simulink subsystem "canStates"  (R2022b)
settings: Solver=VariableStepAuto  StartTime=0.0  StopTime=10.0  RelTol=1e-3
libraries: states_lib x32
settings Model: Creator=serga  LastModifiedBy=serga

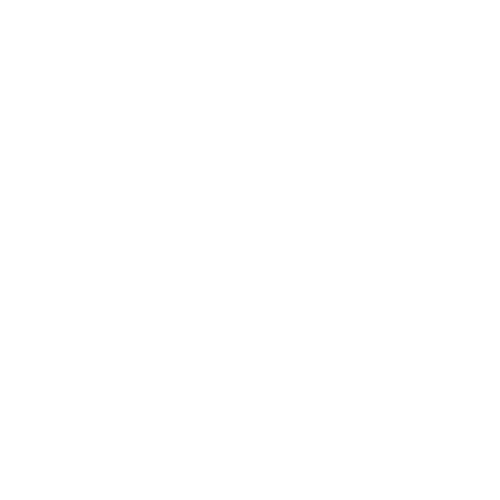
[thumbnail: Simulink's stored preview of the top-level diagram]
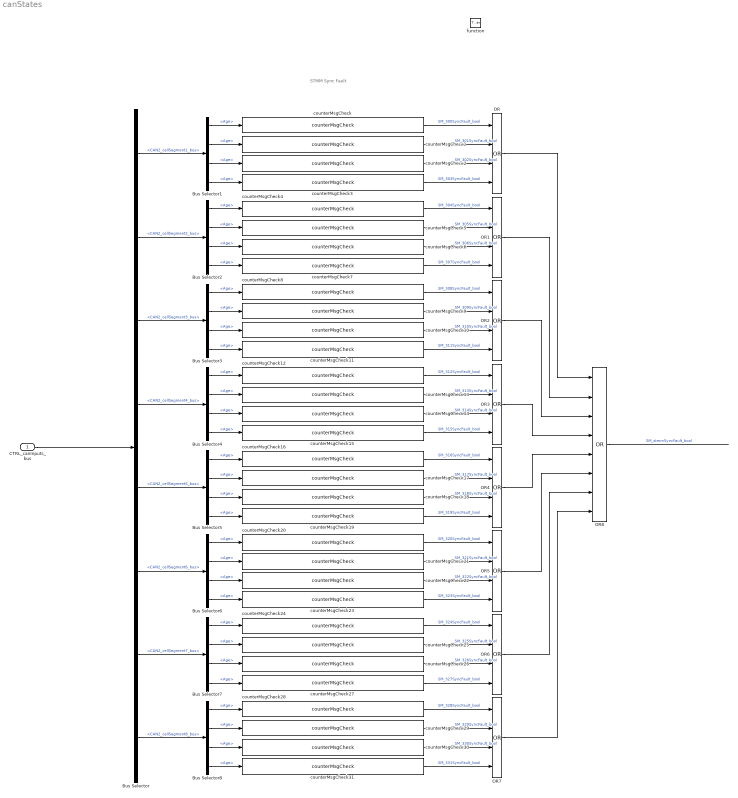
== system canStates ==
  note: STMM Sync Fault
  CTRL_canInputs_bus : Inport
  function : TriggerPort  TriggerType=function-call  VariantControl=(inherit)
  Bus Selector : BusSelector  OutputSignals=IN_can2Inputs_bus.CAN2_stmm_bus.CAN2_cellSegment1_bus,IN_can2Inputs_bus.CAN2_stmm_bus.CAN2_cellSegment2_bus,IN_can2Inputs_bus.CAN2_stmm_bus.CAN2_cellSegment3_bus,IN_can2Inputs_bus.CAN2_stmm_bus.CAN2_cellSegment4_bus,IN_can2Inputs_bus.CAN2_stmm_bus.CAN2_cellSegment5_bus,IN_can2Inputs_bus.CAN2_stmm_bus.CAN2_cellSegment6_bus,IN_can2Inputs_bus.CAN2_stmm_bus.CAN2_cellSegment7_bus,IN_can2Inputs_bus.CAN2_stmm_bus.CAN2_cellSegment8_bus
  Bus Selector1 : BusSelector  OutputSignals=CAN2_stmm_300_bus.Age,CAN2_stmm_301_bus.Age,CAN2_stmm_302_bus.Age,CAN2_stmm_303_bus.Age
  Bus Selector2 : BusSelector  OutputSignals=CAN2_stmm_304_bus.Age,CAN2_stmm_305_bus.Age,CAN2_stmm_306_bus.Age,CAN2_stmm_307_bus.Age
  Bus Selector3 : BusSelector  OutputSignals=CAN2_stmm_308_bus.Age,CAN2_stmm_309_bus.Age,CAN2_stmm_310_bus.Age,CAN2_stmm_311_bus.Age
  Bus Selector4 : BusSelector  OutputSignals=CAN2_stmm_312_bus.Age,CAN2_stmm_313_bus.Age,CAN2_stmm_314_bus.Age,CAN2_stmm_315_bus.Age
  Bus Selector5 : BusSelector  OutputSignals=CAN2_stmm_316_bus.Age,CAN2_stmm_317_bus.Age,CAN2_stmm_318_bus.Age,CAN2_stmm_319_bus.Age
  Bus Selector6 : BusSelector  OutputSignals=CAN2_stmm_320_bus.Age,CAN2_stmm_321_bus.Age,CAN2_stmm_322_bus.Age,CAN2_stmm_323_bus.Age
  Bus Selector7 : BusSelector  OutputSignals=CAN2_stmm_324_bus.Age,CAN2_stmm_325_bus.Age,CAN2_stmm_326_bus.Age,CAN2_stmm_327_bus.Age
  Bus Selector8 : BusSelector  OutputSignals=CAN2_stmm_328_bus.Age,CAN2_stmm_329_bus.Age,CAN2_stmm_330_bus.Age,CAN2_stmm_331_bus.Age
  OR{,1..7} (8 alike) : Logic  Operator=OR  Inputs=4  IconShape=distinctive  AllPortsSameDT=off  OutDataTypeStr=boolean
  OR8 : Logic  Operator=OR  Inputs=8  IconShape=distinctive  AllPortsSameDT=off  OutDataTypeStr=boolean
  counterMsgCheck : states_lib/counterMsgCheck  pos='300'
  counterMsgCheck1 : states_lib/counterMsgCheck  pos='301'
  counterMsgCheck10 : states_lib/counterMsgCheck  pos='310'
  counterMsgCheck11 : states_lib/counterMsgCheck  pos='311'
  counterMsgCheck12 : states_lib/counterMsgCheck  pos='312'
  counterMsgCheck13 : states_lib/counterMsgCheck  pos='313'
  counterMsgCheck14 : states_lib/counterMsgCheck  pos='314'
  counterMsgCheck15 : states_lib/counterMsgCheck  pos='315'
  counterMsgCheck16 : states_lib/counterMsgCheck  pos='316'
  counterMsgCheck17 : states_lib/counterMsgCheck  pos='317'
  counterMsgCheck18 : states_lib/counterMsgCheck  pos='318'
  counterMsgCheck19 : states_lib/counterMsgCheck  pos='319'
  counterMsgCheck2 : states_lib/counterMsgCheck  pos='302'
  counterMsgCheck20 : states_lib/counterMsgCheck  pos='320'
  counterMsgCheck21 : states_lib/counterMsgCheck  pos='321'
  counterMsgCheck22 : states_lib/counterMsgCheck  pos='322'
  counterMsgCheck23 : states_lib/counterMsgCheck  pos='323'
  counterMsgCheck24 : states_lib/counterMsgCheck  pos='324'
  counterMsgCheck25 : states_lib/counterMsgCheck  pos='325'
  counterMsgCheck26 : states_lib/counterMsgCheck  pos='326'
  counterMsgCheck27 : states_lib/counterMsgCheck  pos='327'
  counterMsgCheck28 : states_lib/counterMsgCheck  pos='328'
  counterMsgCheck29 : states_lib/counterMsgCheck  pos='329'
  counterMsgCheck3 : states_lib/counterMsgCheck  pos='303'
  counterMsgCheck30 : states_lib/counterMsgCheck  pos='330'
  counterMsgCheck31 : states_lib/counterMsgCheck  pos='331'
  counterMsgCheck4 : states_lib/counterMsgCheck  pos='304'
  counterMsgCheck5 : states_lib/counterMsgCheck  pos='305'
  counterMsgCheck6 : states_lib/counterMsgCheck  pos='306'
  counterMsgCheck7 : states_lib/counterMsgCheck  pos='307'
  counterMsgCheck8 : states_lib/counterMsgCheck  pos='308'
  counterMsgCheck9 : states_lib/counterMsgCheck  pos='309'
  wires:
  CTRL_canInputs_bus/1 -> Bus Selector/1
  Bus Selector/1 -> Bus Selector1/1  "<CAN2_cellSegment1_bus>"
  Bus Selector1/1 -> counterMsgCheck/1  "<Age>"
  Bus Selector1/2 -> counterMsgCheck1/1  "<Age>"
  Bus Selector1/3 -> counterMsgCheck2/1  "<Age>"
  Bus Selector1/4 -> counterMsgCheck3/1  "<Age>"
  Bus Selector/2 -> Bus Selector2/1  "<CAN2_cellSegment2_bus>"
  Bus Selector2/1 -> counterMsgCheck4/1  "<Age>"
  Bus Selector2/2 -> counterMsgCheck5/1  "<Age>"
  Bus Selector2/3 -> counterMsgCheck6/1  "<Age>"
  Bus Selector2/4 -> counterMsgCheck7/1  "<Age>"
  Bus Selector/3 -> Bus Selector3/1  "<CAN2_cellSegment3_bus>"
  Bus Selector3/1 -> counterMsgCheck8/1  "<Age>"
  Bus Selector3/2 -> counterMsgCheck9/1  "<Age>"
  Bus Selector3/3 -> counterMsgCheck10/1  "<Age>"
  Bus Selector3/4 -> counterMsgCheck11/1  "<Age>"
  Bus Selector/4 -> Bus Selector4/1  "<CAN2_cellSegment4_bus>"
  Bus Selector4/1 -> counterMsgCheck12/1  "<Age>"
  Bus Selector4/2 -> counterMsgCheck13/1  "<Age>"
  Bus Selector4/3 -> counterMsgCheck14/1  "<Age>"
  Bus Selector4/4 -> counterMsgCheck15/1  "<Age>"
  Bus Selector/5 -> Bus Selector5/1  "<CAN2_cellSegment5_bus>"
  Bus Selector5/1 -> counterMsgCheck16/1  "<Age>"
  Bus Selector5/2 -> counterMsgCheck17/1  "<Age>"
  Bus Selector5/3 -> counterMsgCheck18/1  "<Age>"
  Bus Selector5/4 -> counterMsgCheck19/1  "<Age>"
  Bus Selector/6 -> Bus Selector6/1  "<CAN2_cellSegment6_bus>"
  Bus Selector6/1 -> counterMsgCheck20/1  "<Age>"
  Bus Selector6/2 -> counterMsgCheck21/1  "<Age>"
  Bus Selector6/3 -> counterMsgCheck22/1  "<Age>"
  Bus Selector6/4 -> counterMsgCheck23/1  "<Age>"
  Bus Selector7/1 -> counterMsgCheck24/1  "<Age>"
  Bus Selector7/2 -> counterMsgCheck25/1  "<Age>"
  Bus Selector7/3 -> counterMsgCheck26/1  "<Age>"
  Bus Selector7/4 -> counterMsgCheck27/1  "<Age>"
  Bus Selector/7 -> Bus Selector7/1  "<CAN2_cellSegment7_bus>"
  Bus Selector8/1 -> counterMsgCheck28/1  "<Age>"
  Bus Selector8/2 -> counterMsgCheck29/1  "<Age>"
  Bus Selector8/3 -> counterMsgCheck30/1  "<Age>"
  Bus Selector8/4 -> counterMsgCheck31/1  "<Age>"
  Bus Selector/8 -> Bus Selector8/1  "<CAN2_cellSegment8_bus>"
  counterMsgCheck/1 -> OR/1  "SM_300SyncFault_bool"
  counterMsgCheck1/1 -> OR/2  "SM_301SyncFault_bool"
  counterMsgCheck2/1 -> OR/3  "SM_302SyncFault_bool"
  counterMsgCheck3/1 -> OR/4  "SM_303SyncFault_bool"
  counterMsgCheck4/1 -> OR1/1  "SM_304SyncFault_bool"
  counterMsgCheck7/1 -> OR1/4  "SM_307SyncFault_bool"
  counterMsgCheck5/1 -> OR1/2  "SM_305SyncFault_bool"
  counterMsgCheck6/1 -> OR1/3  "SM_306SyncFault_bool"
  counterMsgCheck10/1 -> OR2/3  "SM_310SyncFault_bool"
  counterMsgCheck9/1 -> OR2/2  "SM_309SyncFault_bool"
  counterMsgCheck8/1 -> OR2/1  "SM_308SyncFault_bool"
  counterMsgCheck11/1 -> OR2/4  "SM_311SyncFault_bool"
  counterMsgCheck12/1 -> OR3/1  "SM_312SyncFault_bool"
  counterMsgCheck14/1 -> OR3/3  "SM_314SyncFault_bool"
  counterMsgCheck13/1 -> OR3/2  "SM_313SyncFault_bool"
  counterMsgCheck15/1 -> OR3/4  "SM_315SyncFault_bool"
  counterMsgCheck19/1 -> OR4/4  "SM_319SyncFault_bool"
  counterMsgCheck16/1 -> OR4/1  "SM_316SyncFault_bool"
  counterMsgCheck17/1 -> OR4/2  "SM_317SyncFault_bool"
  counterMsgCheck18/1 -> OR4/3  "SM_318SyncFault_bool"
  counterMsgCheck23/1 -> OR5/4  "SM_323SyncFault_bool"
  counterMsgCheck22/1 -> OR5/3  "SM_322SyncFault_bool"
  counterMsgCheck20/1 -> OR5/1  "SM_320SyncFault_bool"
  counterMsgCheck21/1 -> OR5/2  "SM_321SyncFault_bool"
  counterMsgCheck27/1 -> OR6/4  "SM_327SyncFault_bool"
  counterMsgCheck26/1 -> OR6/3  "SM_326SyncFault_bool"
  counterMsgCheck24/1 -> OR6/1  "SM_324SyncFault_bool"
  counterMsgCheck25/1 -> OR6/2  "SM_325SyncFault_bool"
  counterMsgCheck28/1 -> OR7/1  "SM_328SyncFault_bool"
  counterMsgCheck29/1 -> OR7/2  "SM_329SyncFault_bool"
  counterMsgCheck30/1 -> OR7/3  "SM_330SyncFault_bool"
  counterMsgCheck31/1 -> OR7/4  "SM_331SyncFault_bool"
  OR3/1 -> OR8/4
  OR4/1 -> OR8/5
  OR2/1 -> OR8/3
  OR1/1 -> OR8/2
  OR/1 -> OR8/1
  OR5/1 -> OR8/6
  OR6/1 -> OR8/7
  OR7/1 -> OR8/8
  OR8/1 -> ?  "SM_stmmSyncFault_bool"
